simulink model "Boost_Converter"  (R2020a)
settings: Solver=VariableStepAuto  StartTime=0.0  StopTime=10.0  RelTol=1e-3
libraries: powerlib x14
settings Model: Creator=rajgo  LastModifiedBy=rajgo

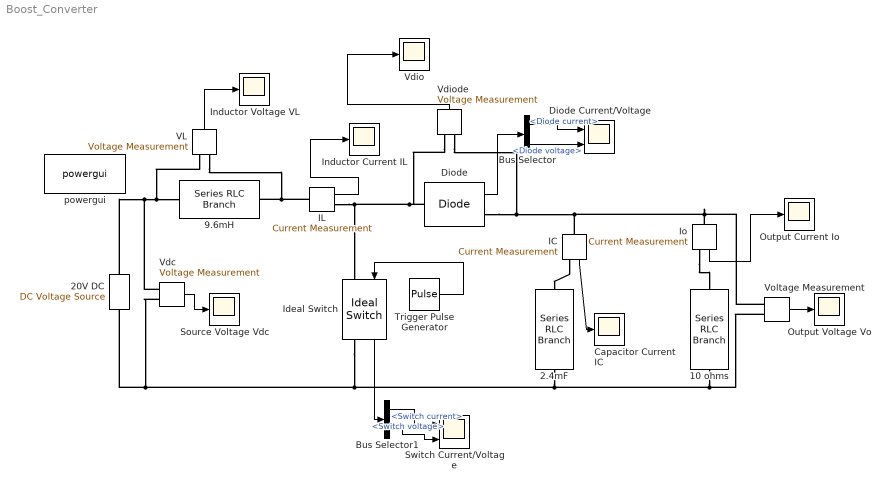
== system Boost_Converter ==
  " Ideal Switch" : powerlib/Power Electronics/Ideal Switch  Ron=0.00000000001  Lon=0  IC=0  Rs=inf  Cs=inf  Measurements=on
  10 ohms : powerlib/Elements/Series RLC Branch  LConnTagsString=__new0  RConnTagsString=__new0  BranchType=R  Resistance=10  Inductance=1e-3  SetiL0=off  InitialCurrent=0  Capacitance=1e-6  Setx0=off  InitialVoltage=0  Measurements=None
  2.4mF : powerlib/Elements/Series RLC Branch  LConnTagsString=__new0  RConnTagsString=__new0  BranchType=C  Resistance=1  Inductance=1e-3  SetiL0=off  InitialCurrent=0  Capacitance=2.4e-3  Setx0=off  InitialVoltage=0  Measurements=None
  20V DC : powerlib/Electrical Sources/DC Voltage Source  Amplitude=20  Measurements=None
  9.6mH : powerlib/Elements/Series RLC Branch  LConnTagsString=__new0  RConnTagsString=__new0  BranchType=L  Resistance=1  Inductance=9.6e-3  SetiL0=off  InitialCurrent=0  Capacitance=1e-6  Setx0=off  InitialVoltage=0  Measurements=None
  Bus Selector : BusSelector  OutputSignals=Diode current,Diode voltage
  Bus Selector1 : BusSelector  OutputSignals=Switch current,Switch voltage
  Capacitor Current IC : Scope
  "Diode " : powerlib/Power Electronics/Diode  Ron=0.000000000000001  Lon=0  Vf=0  IC=0  UseSnubber=0  Rs=inf  Cs=0  Measurements=on
  Diode Current/Voltage : Scope  NumInputPorts=2
  IC : powerlib/Measurements/Current Measurement  PhasorSimulation=off  OutputType=Complex  PSBequivalent=0
  IL : powerlib/Measurements/Current Measurement  PhasorSimulation=off  OutputType=Complex  PSBequivalent=0
  Inductor Current IL : Scope
  Inductor Voltage VL : Scope
  Io : powerlib/Measurements/Current Measurement  PhasorSimulation=off  OutputType=Complex  PSBequivalent=0
  Output Current Io : Scope
  Output Voltage Vo : Scope
  Source Voltage Vdc : Scope
  Switch Current/Voltage : Scope  NumInputPorts=2
  Trigger Pulse Generator : DiscretePulseGenerator  PulseType=Time based  Amplitude=10  Period=1/5000  PulseWidth=60
  VL : powerlib/Measurements/Voltage Measurement  PhasorSimulation=off  OutputType=Complex  PSBequivalent=0
  Vdc : powerlib/Measurements/Voltage Measurement  PhasorSimulation=off  OutputType=Complex  PSBequivalent=0
  Vdio : Scope
  Vdiode : powerlib/Measurements/Voltage Measurement  PhasorSimulation=off  OutputType=Complex  PSBequivalent=0
  Voltage Measurement : powerlib/Measurements/Voltage Measurement  PhasorSimulation=off  OutputType=Complex  PSBequivalent=0
  powergui : powerlib/powergui  Priority=1  SimulationMode=Continuous  SampleTime=50e-6  frequency=60  Iterations=50  frequencyindice=0  Pbase=100e6  ErrMax=1e-4  UnitsV=kV  UnitsW=MW  buscounter=0  FunctionMessages=off  echomessages=off  EnableUseOfTLC=off  CurrentSourceSwitches=off  DisableSnubberDevices=off  DisableRonSwitches=off  DisableVfSwitches=off  DisplayEquations=off  AutomaticDiscreteSolvers=off  SolverType=Tustin/Backward Euler (TBE)  Interpol=off  ExternalGateDelay=off  methode=off  Ts=100  x0status=blocks  SPID=on  SwTol=0  HookPort=off  NonlinearTolerance=1e-4  nMaxIteration=100  ContinueOnMaxIteration=off  RestoreLinks=warning  ResistiveCurrentMeasurement=off  Frange=[0:2:500]  Ylog=off  Xlog=on  ShowGrid=off  save=off  variable=ZData  structure=0  ZoomFFT=off  StartTime=0.0  cycles=1  DisplayStyle=1  fundamental=60  FreqAxis=off  MaxFrequency=1000  frequencyindicesteady=1  RmsSteady=1  display=off
  wires:
  Trigger Pulse Generator/1 -> " Ideal Switch"/1
  Voltage Measurement/1 -> Output Voltage Vo/1
  Vdc/1 -> Source Voltage Vdc/1
  IL/1 -> Inductor Current IL/1
  "Diode "/1 -> Bus Selector/1
  Bus Selector/1 -> Diode Current/Voltage/1  "<Diode current>"
  Bus Selector/2 -> Diode Current/Voltage/2  "<Diode voltage>"
  IC/1 -> Capacitor Current IC/1
  Io/1 -> Output Current Io/1
  VL/1 -> Inductor Voltage VL/1
  " Ideal Switch"/1 -> Bus Selector1/1
  Bus Selector1/1 -> Switch Current/Voltage/1  "<Switch current>"
  Bus Selector1/2 -> Switch Current/Voltage/2  "<Switch voltage>"
  Vdiode/1 -> Vdio/1
  connections:
  20V DC/RConn1 -- 9.6mH/LConn1 -- VL/LConn1 -- Vdc/LConn1
  "Diode "/LConn1 -- IL/RConn1 -- " Ideal Switch"/LConn1 -- Vdiode/LConn1
  " Ideal Switch"/RConn1 -- 10 ohms/RConn1 -- Voltage Measurement/LConn2 -- 2.4mF/RConn1 -- Vdc/LConn2 -- 20V DC/LConn1
  "Diode "/RConn1 -- Vdiode/LConn2 -- Io/LConn1 -- Voltage Measurement/LConn1 -- IC/LConn1
  IL/LConn1 -- VL/LConn2 -- 9.6mH/RConn1
  IC/RConn1 -- 2.4mF/LConn1
  Io/RConn1 -- 10 ohms/LConn1
